simulink model "xpccanintpc104"  (Simulink 4.00)
settings: Solver=FixedStepDiscrete  StartTime=0.0  StopTime=300  RelTol=1e-3
undefined symbols (not defined in the file or in its folder): bit, Standard
libraries: xpclib x8, simulink3 x1
settings Model: Creator=mvetsch  LastModifiedBy=rroy  RTWSystemTargetFile=xpctarget.tlc  RTWOptions="-aEnforceIntegerDowncast=1 -aExtMode=1 -aFoldNonRolledExpr=1 -aForceParamTrailComments=0 -aGenerateComments=1 -aIncHierarchyInIds=0 -aInlineInvariantSignals=0 -aInlineParameters=0 -aLocalBlockOutputs=0 -aRL32IRQSourceModifier=\"Timer\" -aRL32LogBufSizeModifier=100000 -aRL32LogTETModifier=1 -aRL32ModeModifier=\"Real-Time\" -aRL32ObjectName=\"tg\" -aRL32ScopeModifier=1 -aRTWVerbose=1 -aRollThreshold=5 -aShowEliminatedStatements=1"  RTWTemplateMakefile=xpc_default_tmf  ExtModeMexFile=ext_xpc  ExtModeArmWhenConnect=off  OptimizeBlockIOStorage=off  BlockReductionOpt=off

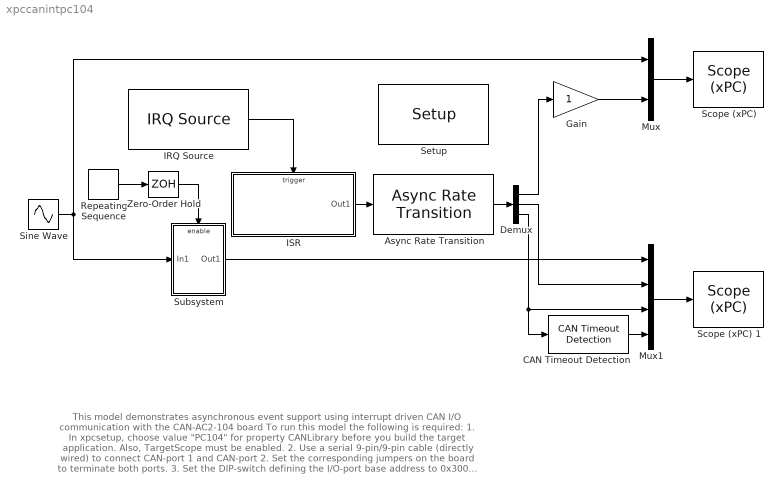
== system xpccanintpc104 ==
  note: This model demonstrates asynchronous event support using interrupt driven CAN I/O communication
      | with the CAN-AC2-104 board
      |
      | To run this model the following is required:
      |
      | 1. In xpcsetup, choose value "PC104" for property CANLibrary before you build the
      | target application. Also, TargetScope must be enabled.
      |
      | 2. Use a serial 9-pin/9-pin cable (directly wired) to connect CAN-port 1 and CAN-port 2.
      | Set the corresponding jumpers on the board to terminate both ports.
      |
      | 3. Set the DIP-switch defining the I/O-port base address to 0x300 (hex)
      |
      | 4. Make sure that IRQ line 5 is assigned only to the CAN-AC2-104 board.
      | To assure this, reserve IRQ 5 in the target machine BIOS setup as being
      | used by a legacy ISA device. Then build the target application.
  Async Rate Transition : xpclib/Asynchronous Event/Async Rate Transition  sample_time=0.01
  CAN Timeout Detection : xpclib/CAN/Utilities/CAN Timeout Detection  AncestorBlock=xpclib_pc104/CAN/Utilities/CAN Timeout Detection  timeout=0.02
  Demux : Demux  Outputs=3  BusSelectionMode=off
  Gain : Gain  Gain=1  Multiplication=Element-wise(K.*u)  SaturateOnIntegerOverflow=on
  IRQ Source : xpclib/Asynchronous Event/IRQ Source  irqNo=5  preempt=on  b_type=Softing CAN-AC2-104  slot=-1
  ISR : Subsystem  TreatAsAtomicUnit=on
      settings: RTWFcnNameOpts=Auto  RTWFileNameOpts=Auto
  Mux : Mux  Inputs=2
  Mux1 : Mux  Inputs=4
  Repeating Sequence : simulink3/Sources/Repeating Sequence  rep_seq_t=[0,2,2.01,4]  rep_seq_y=[1,1,0,0]
  "Scope (xPC) " : xpclib/Misc./Scope (xPC)   scopeno=1  scopetype=Target  viewmode=Graphical rolling  grid=on  ylimits=[0,0]  autostart=on  nosamples=250  noprepostsamples=0  interleave=1  triggermode=FreeRun  triggersignal=1  triggerlevel=0.0  triggerslope=either  triggerscope=1
  Scope (xPC) 1 : xpclib/Misc./Scope (xPC)   scopeno=2  scopetype=Target  viewmode=Numerical  grid=on  ylimits=[0,0]  autostart=on  nosamples=10  noprepostsamples=0  interleave=1  triggermode=FreeRun  triggersignal=1  triggerlevel=0.0  triggerslope=either  triggerscope=1
  "Setup " : xpclib/CAN/Softing/CAN-AC2-104 SJA 1000/Setup   board=1  can1Baudrate=1 MBaud  can1UserBR=[1,1,4,3]  can2Baudrate=1 MBaud  can2UserBR=[1,1,4,3]  init=[]  term=[]  ioBaseAddressL=0x300  memBaseAddressL=0xd0000  intNo=5
  Sine Wave : Sin  SineType=Time-based  Amplitude=1  Bias=0  Frequency=5  Phase=0  Samples=10  SampleTime=0.01  Offset=0
  Subsystem : Subsystem  TreatAsAtomicUnit=on
      settings: RTWFcnNameOpts=Auto  RTWFileNameOpts=Auto
  Zero-Order Hold : ZeroOrderHold  SampleTime=0.01
  wires:
  Sine Wave/1 -> Mux/1, Subsystem/1(In1)
  ISR/1(Out1) -> Async Rate Transition/1
  Demux/1 -> Gain/1
  Gain/1 -> Mux/2
  Mux/1 -> "Scope (xPC) "/1
  Mux1/1 -> Scope (xPC) 1/1
  Demux/3 -> Mux1/3, CAN Timeout Detection/1
  Demux/2 -> Mux1/2
  CAN Timeout Detection/1 -> Mux1/4
  Subsystem/1(Out1) -> Mux1/1
  Repeating Sequence/1 -> Zero-Order Hold/1
  IRQ Source/1 -> ISR/Trigger
  Async Rate Transition/1 -> Demux/1
  Zero-Order Hold/1 -> Subsystem/Enable

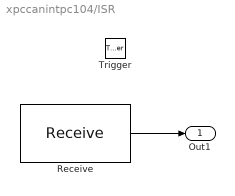
== system xpccanintpc104/ISR ==
  Trigger : TriggerPort  TriggerType=function-call  OutputDataType=auto
  "Receive " : xpclib/CAN/Softing/CAN-AC2-104 SJA 1000/Receive   board=1  canPort=CAN 2  range=Standard (11-bit)  ids=[50]  output=Data - Status - Timestamp  inten=on  ts=-1  ididx=[0]
  Out1 : Outport  Port=1
  wires:
  "Receive "/1 -> Out1/1

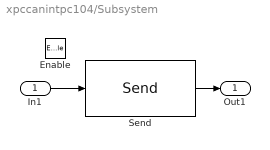
== system xpccanintpc104/Subsystem ==
  In1 : Inport  Port=1  LatchInput=off
  Enable : EnablePort  StatesWhenEnabling=reset
  "Send " : xpclib/CAN/Softing/CAN-AC2-104 SJA 1000/Send   board=1  canPort=CAN 1  range=Standard (11-bit)  ids=[50]  sizes=[8]  output=on  ts=0.01  ididx=[0]
  Out1 : Outport  Port=1  OutputWhenDisabled=reset  InitialOutput=0
  wires:
  In1/1 -> "Send "/1
  "Send "/1 -> Out1/1
